simulink model "DualStreamSSR"  (R2020a)
settings: Solver=VariableStepAuto  StartTime=0.0  StopTime=4096  RelTol=1e-3
PreLoadFcn:
  | SSR4_init
InitFcn:
  | SSR4_init
values from neighbouring files (symbols this model uses):
  N = 8    [SSR4_init.m]
  SHIFT_ACC = 15    [SSR4_init.m]
  Taps = NormalizeCoef(UTaps,32768)    [SSR4_init.m]
undefined symbols (not defined in the file or in its folder): DoubleStream, FIR_MultiKernel_cin, FIR_MultiKernel_cincout, FIR_MultiKernel_cout, xc7vx485tffg1157
libraries: ModelComposer x129, dspsrcs4 x1, simulink x1
(part 5 of 5)

== matlab function DualStreamSSR/ComplexSource4/MATLAB Function ==
  data: u input; y1 output; y2 output; y3 output; y4 output; y5 output; y6 output; y7 output; y8 output; y9 output; y10 output; y11 output; y12 output; y13 output; y14 output; y15 output; y16 output
function [y1,y2,y3,y4,y5,y6,y7,y8,y9,y10,y11,y12,y13,y14,y15,y16] = fcn(u)
[y1,y2] = CreateStreams(u(1:8:end));
[y3,y4] = CreateStreams(u(2:8:end));
[y5,y6] = CreateStreams(u(3:8:end));
[y7,y8] = CreateStreams(u(4:8:end));
[y9,y10] = CreateStreams(u(5:8:end));
[y11,y12] = CreateStreams(u(6:8:end));
[y13,y14] = CreateStreams(u(7:8:end));
[y15,y16] = CreateStreams(u(8:8:end));
end
function [s1, s2] = CreateStreams(p)
L = length(p);
p = reshape(p,4,L/4);
s1 = reshape(p(:,1:2:L/4),1,L/2);
s2 = reshape(p(:,2:2:L/4),1,L/2);
end
